simulink model "Einfache_Zustandsrueckfuehrung_linear"  (R2021b)
settings: Solver=FixedStepAuto  StartTime=0.0  StopTime=10  FixedStep=1/1e4  RelTol=1e-3
undefined symbols (not defined in the file): A, B, C, d, k_LMI_1, x_Ruhe
settings Model: Creator=basti  LastModifiedBy=basti

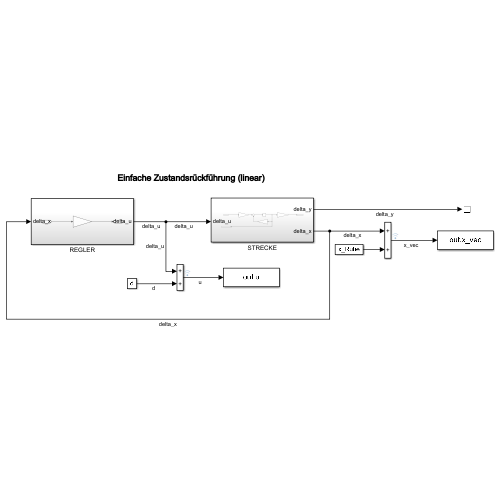
[thumbnail: Simulink's stored preview of the top-level diagram]
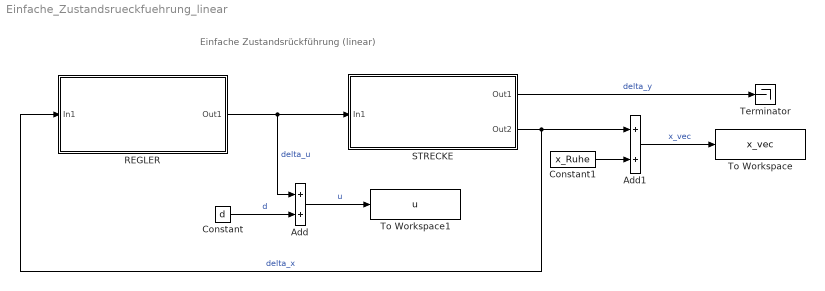
== system Einfache_Zustandsrueckfuehrung_linear ==
  note: Einfache Zustandsrückführung (linear)
  Add : Sum
  Add1 : Sum
  Constant : Constant  Value=d
  Constant1 : Constant  Value=x_Ruhe
  REGLER : Subsystem
  STRECKE : Subsystem
  Terminator : Terminator
  To Workspace : ToWorkspace  VariableName=x_vec  SaveFormat=Timeseries  SampleTime=-1
  To Workspace1 : ToWorkspace  VariableName=u  SaveFormat=Timeseries  SampleTime=-1
  wires:
  STRECKE/2(Out2) -> REGLER/1(In1), Add1/1  "delta_x"
  STRECKE/1(Out1) -> Terminator/1  "delta_y"
  Constant1/1 -> Add1/2
  Add1/1 -> To Workspace/1  "x_vec"
  Constant/1 -> Add/2  "d"
  REGLER/1(Out1) -> Add/1, STRECKE/1(In1)  "delta_u"
  Add/1 -> To Workspace1/1  "u"

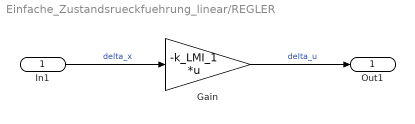
== system Einfache_Zustandsrueckfuehrung_linear/REGLER ==
  In1 : Inport
  Gain : Gain  Gain=-k_LMI_1  Multiplication=Matrix(K*u) (u vector)
  Out1 : Outport
  wires:
  In1/1 -> Gain/1  "delta_x"
  Gain/1 -> Out1/1  "delta_u"

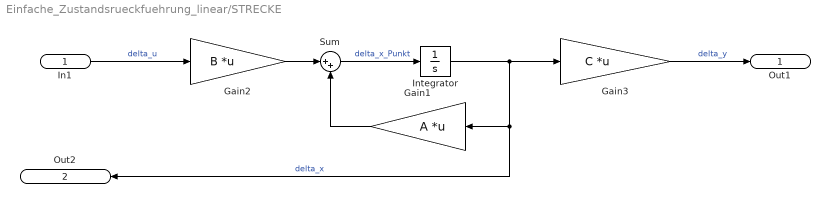
== system Einfache_Zustandsrueckfuehrung_linear/STRECKE ==
  In1 : Inport
  Gain1 : Gain  Gain=A  Multiplication=Matrix(K*u) (u vector)
  Gain2 : Gain  Gain=B  Multiplication=Matrix(K*u) (u vector)
  Gain3 : Gain  Gain=C  Multiplication=Matrix(K*u) (u vector)
  Integrator : Integrator  InitialCondition=[-10; 0]
  Sum : Sum  Inputs=|++
  Out1 : Outport
  Out2 : Outport  Port=2
  wires:
  Gain1/1 -> Sum/2
  Gain3/1 -> Out1/1  "delta_y"
  Sum/1 -> Integrator/1  "delta_x_Punkt"
  Integrator/1 -> Gain3/1, Out2/1, Gain1/1  "delta_x"
  Gain2/1 -> Sum/1
  In1/1 -> Gain2/1  "delta_u"
